simulink model "MagNoiseTest"  (R2022b)
settings: Solver=ode4  StartTime=0.0  StopTime=6000  FixedStep=dm.dt  RelTol=1e-3
InitFcn:
  | Tu = 210; %s
  | Wu   = 2*pi/Tu;
  | Zeta = 0.707;
  | SOFC = tf(Wu^2,[1 2*Zeta*Wu Wu^2]);
  | SOFD = c2d(SOFC, fsw.bdot_period);
undefined symbols (not defined in the file or in its folder): dm
libraries: aerolibtransform2 x1
settings Model: VariantFading=off  Creator=USER  LastModifiedBy=Jack-STK2

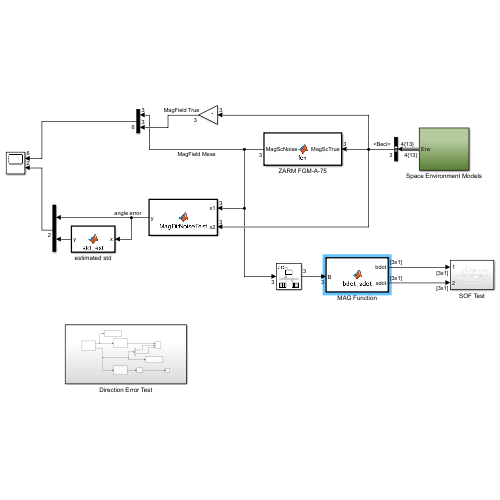
[thumbnail: Simulink's stored preview of the top-level diagram]
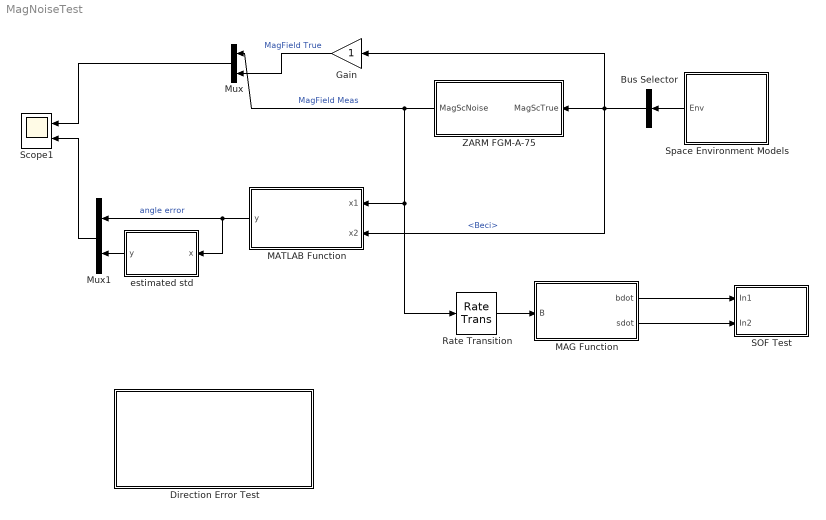
== system MagNoiseTest ==
  Bus Selector : BusSelector  OutputSignals=Beci
  Direction Error Test : Subsystem
  Gain : Gain
  MAG Function : MATLAB Function  TreatAsAtomicUnit=on
  MATLAB Function : MATLAB Function  TreatAsAtomicUnit=on
  Mux : Mux  Inputs=2
  Mux1 : Mux  Inputs=2
  Rate Transition : RateTransition  InitialCondition=zeros(3,1)  OutPortSampleTime=fsw.bdot_period
  SOF Test : Subsystem
  Scope1 : Scope  NumInputPorts=2
  Space Environment Models : Subsystem
  ZARM FGM-A-75 : MATLAB Function  TreatAsAtomicUnit=on
  estimated std : MATLAB Function  TreatAsAtomicUnit=on
  wires:
  Space Environment Models/1(Env) -> Bus Selector/1
  Bus Selector/1 -> ZARM FGM-A-75/1(MagScTrue), Gain/1, MATLAB Function/2(x2)  "<Beci>"
  ZARM FGM-A-75/1(MagScNoise) -> MATLAB Function/1(x1), Rate Transition/1, Mux/1  "MagField Meas"
  MATLAB Function/1(y) -> estimated std/1(x), Mux1/1  "angle error"
  Mux/1 -> Scope1/1
  Gain/1 -> Mux/2  "MagField True"
  estimated std/1(y) -> Mux1/2
  Mux1/1 -> Scope1/2
  Rate Transition/1 -> MAG Function/1(B)
  MAG Function/1(bdot) -> SOF Test/1(In1)
  MAG Function/2(sdot) -> SOF Test/2(In2)

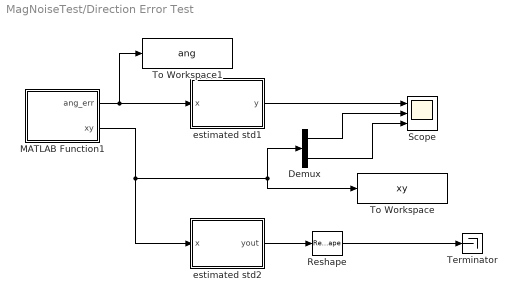
== system MagNoiseTest/Direction Error Test ==
  Demux : Demux  Outputs=2
  MATLAB Function1 : MATLAB Function  TreatAsAtomicUnit=on
  Reshape : Reshape
  Scope : Scope  NumInputPorts=3
  Terminator : Terminator
  To Workspace : ToWorkspace  VariableName=xy  SaveFormat=Timeseries  SampleTime=-1
      settings: Save2DSignal=2-D array (concatenate along first dimension)
  To Workspace1 : ToWorkspace  VariableName=ang  SaveFormat=Timeseries  SampleTime=-1
  estimated std1 : MATLAB Function  TreatAsAtomicUnit=on
  estimated std2 : MATLAB Function  TreatAsAtomicUnit=on
  wires:
  Demux/2 -> Scope/3
  MATLAB Function1/1(ang_err) -> To Workspace1/1, estimated std1/1(x)
  Demux/1 -> Scope/2
  estimated std2/1(yout) -> Reshape/1
  Reshape/1 -> Terminator/1
  MATLAB Function1/2(xy) -> Demux/1, To Workspace/1, estimated std2/1(x)
  estimated std1/1(y) -> Scope/1

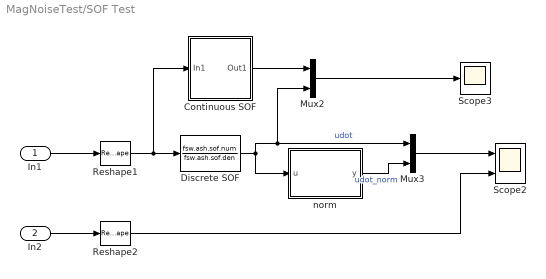
== system MagNoiseTest/SOF Test ==
  In1 : Inport
  In2 : Inport  Port=2
  Continuous SOF : Subsystem
  Discrete SOF : DiscreteTransferFcn  Numerator=fsw.ash.sof.num  Denominator=fsw.ash.sof.den
  Mux2 : Mux  Inputs=2
  Mux3 : Mux  Inputs=2
  Reshape1 : Reshape
  Reshape2 : Reshape
  Scope2 : Scope  NumInputPorts=2
  Scope3 : Scope
  norm : MATLAB Function  TreatAsAtomicUnit=on
  wires:
  Continuous SOF/1(Out1) -> Mux2/1
  Mux3/1 -> Scope2/1
  norm/1(y) -> Mux3/2  "udot_norm"
  Discrete SOF/1 -> norm/1(u), Mux2/2, Mux3/1  "udot"
  Mux2/1 -> Scope3/1
  Reshape1/1 -> Continuous SOF/1(In1), Discrete SOF/1
  Reshape2/1 -> Scope2/2
  In1/1 -> Reshape1/1
  In2/1 -> Reshape2/1

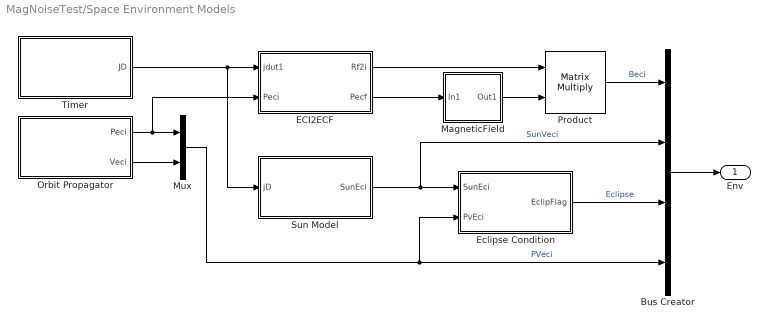
== system MagNoiseTest/Space Environment Models ==
  Bus Creator : BusCreator  Inputs=4
  ECI2ECF : MATLAB Function  TreatAsAtomicUnit=on
  Eclipse Condition : MATLAB Function  TreatAsAtomicUnit=on
  MagneticField : Subsystem
  Mux : Mux  Inputs=2
  "Orbit Propagator " : Subsystem
  Product : Product  Multiplication=Matrix(*)
  Sun Model : MATLAB Function  TreatAsAtomicUnit=on
  Timer : Subsystem
  Env : Outport  VectorParamsAs1DForOutWhenUnconnected=off
  wires:
  ECI2ECF/1(Rf2i) -> Product/1
  Product/1 -> Bus Creator/1  "Beci"
  "Orbit Propagator "/1(Peci) -> ECI2ECF/2(Peci), Mux/1
  "Orbit Propagator "/2(Veci) -> Mux/2
  Timer/1(JD) -> Sun Model/1(jD), ECI2ECF/1(jdut1)
  Mux/1 -> Eclipse Condition/2(PvEci), Bus Creator/4  "PVeci"
  Bus Creator/1 -> Env/1
  Sun Model/1(SunEci) -> Bus Creator/2, Eclipse Condition/1(SunEci)  "SunVeci"
  Eclipse Condition/1(EclipFlag) -> Bus Creator/3  "Eclipse"
  ECI2ECF/2(Pecf) -> MagneticField/1(In1)
  MagneticField/1(Out1) -> Product/2

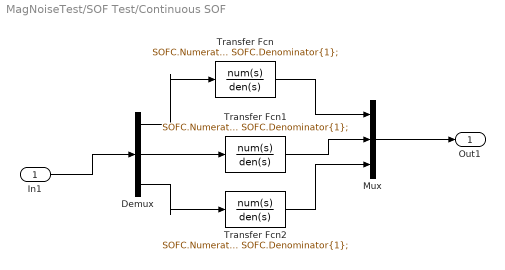
== system MagNoiseTest/SOF Test/Continuous SOF ==
  In1 : Inport
  Demux : Demux  Outputs=3
  Mux : Mux  Inputs=3
  Transfer Fcn : TransferFcn  Numerator=SOFC.Numerator{1}  Denominator=SOFC.Denominator{1};
  Transfer Fcn1 : TransferFcn  Numerator=SOFC.Numerator{1}  Denominator=SOFC.Denominator{1};
  Transfer Fcn2 : TransferFcn  Numerator=SOFC.Numerator{1}  Denominator=SOFC.Denominator{1};
  Out1 : Outport
  wires:
  In1/1 -> Demux/1
  Demux/1 -> Transfer Fcn/1
  Demux/2 -> Transfer Fcn1/1
  Demux/3 -> Transfer Fcn2/1
  Transfer Fcn/1 -> Mux/1
  Transfer Fcn1/1 -> Mux/2
  Transfer Fcn2/1 -> Mux/3
  Mux/1 -> Out1/1

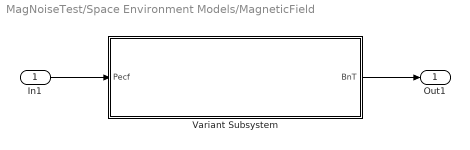
== system MagNoiseTest/Space Environment Models/MagneticField ==
  In1 : Inport
  Variant Subsystem : Subsystem  Variant=on
  Out1 : Outport
  wires:
  In1/1 -> Variant Subsystem/1(Pecf)
  Variant Subsystem/1(BnT) -> Out1/1

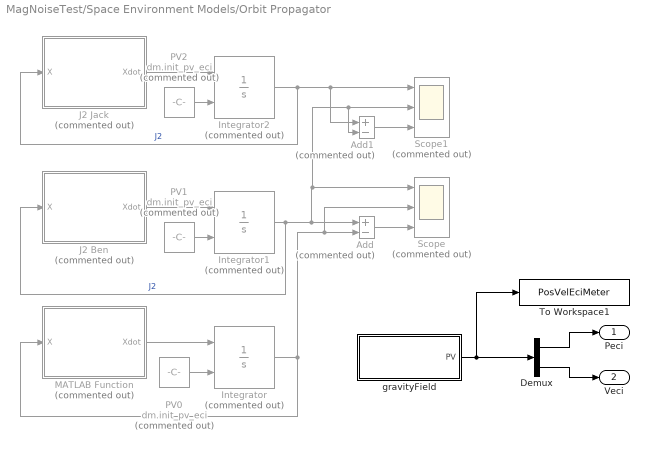
== system MagNoiseTest/Space Environment Models/Orbit Propagator  ==
  Add : Sum  Commented=on  Inputs=+-
  Add1 : Sum  Commented=on  Inputs=+-
  Demux : Demux  Outputs=2
  Integrator : Integrator  Commented=on  InitialConditionSource=external
  Integrator1 : Integrator  Commented=on  InitialConditionSource=external
  Integrator2 : Integrator  Commented=on  InitialConditionSource=external
  J2 Ben : MATLAB Function  Commented=on  TreatAsAtomicUnit=on
  J2 Jack : MATLAB Function  Commented=on  TreatAsAtomicUnit=on
  MATLAB Function : MATLAB Function  Commented=on  TreatAsAtomicUnit=on
  PV0 : Constant  Commented=on  Value=dm.init_pv_eci
  PV1 : Constant  Commented=on  Value=dm.init_pv_eci
  PV2 : Constant  Commented=on  Value=dm.init_pv_eci
  Scope : Scope  Commented=on  NumInputPorts=3
  Scope1 : Scope  Commented=on  NumInputPorts=3
  To Workspace1 : ToWorkspace  VariableName=PosVelEciMeter  SaveFormat=Timeseries  SampleTime=-1
  gravityField : Subsystem  Variant=on
  Peci : Outport  VectorParamsAs1DForOutWhenUnconnected=off
  Veci : Outport  Port=2  VectorParamsAs1DForOutWhenUnconnected=off
  wires:
  Demux/2 -> Veci/1
  MATLAB Function/1(Xdot) -> Integrator/1
  Integrator/1 -> Add/2, Scope/2, MATLAB Function/1(X)
  Demux/1 -> Peci/1
  PV0/1 -> Integrator/2
  PV1/1 -> Integrator1/2
  J2 Ben/1(Xdot) -> Integrator1/1
  Integrator1/1 -> J2 Ben/1(X), Add/1, Add1/2, Scope1/2, Scope/1  "J2"
  Add/1 -> Scope/3
  PV2/1 -> Integrator2/2
  J2 Jack/1(Xdot) -> Integrator2/1
  Integrator2/1 -> J2 Jack/1(X), Add1/1, Scope1/1  "J2"
  Add1/1 -> Scope1/3
  gravityField/1(PV) -> To Workspace1/1, Demux/1

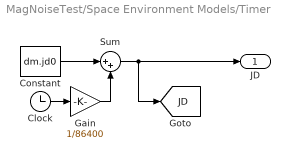
== system MagNoiseTest/Space Environment Models/Timer ==
  Clock : Clock
  Constant : Constant  Value=dm.jd0
  Gain : Gain  Gain=1/86400
  Sum : Sum  Inputs=|++
  JD : Outport  VectorParamsAs1DForOutWhenUnconnected=off
  tag scope: JD=global
  wires:
  Clock/1 -> Gain/1
  Gain/1 -> Sum/2
  Constant/1 -> Sum/1
  Sum/1 -> [JD], JD/1

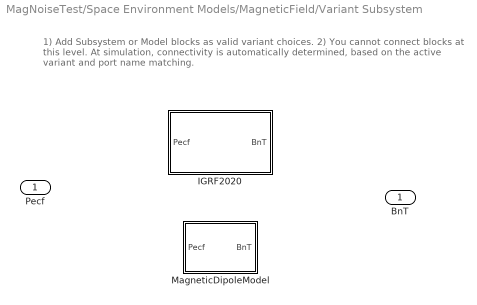
== system MagNoiseTest/Space Environment Models/MagneticField/Variant Subsystem ==
  note: 1) Add Subsystem or Model blocks as valid variant choices.
      | 2) You cannot connect blocks at this level. At simulation, connectivity is automatically
      | determined, based on the active variant and port name matching.
  Pecf : Inport
  IGRF2020 : Subsystem  VariantControl=M_IGRF
  MagneticDipoleModel : MATLAB Function  TreatAsAtomicUnit=on  VariantControl=M_DIPOLE
  BnT : Outport

== system MagNoiseTest/Space Environment Models/Orbit Propagator /gravityField ==
  note: 1) Add Subsystem or Model blocks as valid variant choices.
      | 2) You cannot connect blocks at this level. At simulation, connectivity is automatically
      | determined, based on the active variant and port name matching.
  J2 : Subsystem  VariantControl=G_J2
  TwoBodyRHS : Subsystem  VariantControl=G_TwoBody
  PV : Outport

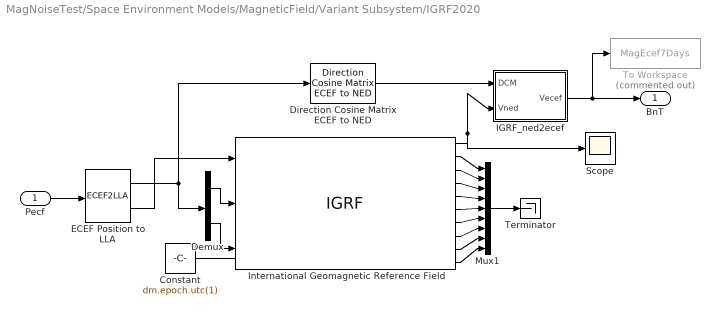
== system MagNoiseTest/Space Environment Models/MagneticField/Variant Subsystem/IGRF2020 ==
  Pecf : Inport
  Constant : Constant  Value=dm.epoch.utc(1)
  Demux : Demux  Outputs=2
  Direction Cosine Matrix ECEF to NED : aerolibtransform2/Direction Cosine Matrix ECEF to NED
  ECEF Position to LLA : ECEF2LLA  R=6378137
  IGRF_ned2ecef : MATLAB Function  TreatAsAtomicUnit=on
  International Geomagnetic Reference Field : IGRF  time_in=off  month=June  day=21  year=2023
      settings: AttributesFormatString=%<generation>
  Mux1 : Mux  Inputs=9
  Scope : Scope
  Terminator : Terminator
  To Workspace : ToWorkspace  Commented=on  VariableName=MagEcef7Days  SaveFormat=Timeseries  SampleTime=-1
  BnT : Outport  VectorParamsAs1DForOutWhenUnconnected=off
  wires:
  International Geomagnetic Reference Field/7 -> Mux1/6
  International Geomagnetic Reference Field/4 -> Mux1/3
  International Geomagnetic Reference Field/3 -> Mux1/2
  International Geomagnetic Reference Field/6 -> Mux1/5
  International Geomagnetic Reference Field/5 -> Mux1/4
  International Geomagnetic Reference Field/9 -> Mux1/8
  International Geomagnetic Reference Field/8 -> Mux1/7
  International Geomagnetic Reference Field/10 -> Mux1/9
  Pecf/1 -> ECEF Position to LLA/1
  Mux1/1 -> Terminator/1
  International Geomagnetic Reference Field/2 -> Mux1/1
  ECEF Position to LLA/1 -> Demux/1, Direction Cosine Matrix ECEF to NED/1
  ECEF Position to LLA/2 -> International Geomagnetic Reference Field/1
  Constant/1 -> ?
  Demux/1 -> International Geomagnetic Reference Field/2
  Demux/2 -> International Geomagnetic Reference Field/3
  Direction Cosine Matrix ECEF to NED/1 -> IGRF_ned2ecef/1(DCM)
  IGRF_ned2ecef/1(Vecef) -> To Workspace/1, BnT/1
  International Geomagnetic Reference Field/1 -> IGRF_ned2ecef/2(Vned), Scope/1

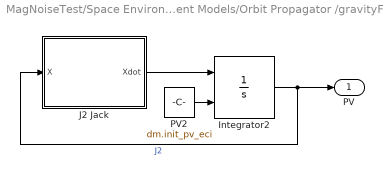
== system MagNoiseTest/Space Environment Models/Orbit Propagator /gravityField/J2 ==
  Integrator2 : Integrator  InitialConditionSource=external
  J2 Jack : MATLAB Function  TreatAsAtomicUnit=on
  PV2 : Constant  Value=dm.init_pv_eci
  PV : Outport
  wires:
  Integrator2/1 -> PV/1, J2 Jack/1(X)  "J2"
  J2 Jack/1(Xdot) -> Integrator2/1
  PV2/1 -> Integrator2/2

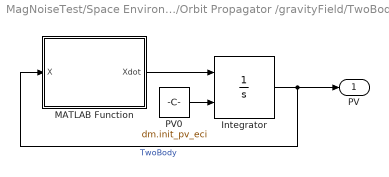
== system MagNoiseTest/Space Environment Models/Orbit Propagator /gravityField/TwoBodyRHS ==
  Integrator : Integrator  InitialConditionSource=external
  MATLAB Function : MATLAB Function  TreatAsAtomicUnit=on
  PV0 : Constant  Value=dm.init_pv_eci
  PV : Outport
  wires:
  Integrator/1 -> PV/1, MATLAB Function/1(X)  "TwoBody"
  MATLAB Function/1(Xdot) -> Integrator/1
  PV0/1 -> Integrator/2

== matlab function MagNoiseTest/Space Environment Models/Sun Model ==
  data: jD input; SunEci output
function SunEci = SunModel(jD)
T = JDCentury(jD);
lamda_mean     = rem(280.460+36000.771*T,360);
mean_anomaly   = rem(357.5291092+35999.05034*T,360);
lamda_ecliptic = lamda_mean+ 1.914666471*sind(mean_anomaly)...
                 + 0.019994643*sind(2*mean_anomaly);
% Obliquity of ecliptic
epsilon = 23.439291 -0.0130042*T;
SunEci  = [cosd(lamda_ecliptic);...
           cosd(epsilon)*sind(lamda_ecliptic);...
           sind(epsilon)*sind(lamda_ecliptic)];

== matlab function MagNoiseTest/Space Environment Models/MagneticField/Variant Subsystem/IGRF2020/IGRF_ned2ecef ==
  data: DCM input; Vecef output; Vned input
function Vecef = fcn(DCM,Vned)

Vecef = DCM'*Vned;

== matlab function MagNoiseTest/Space Environment Models/ECI2ECF ==
  data: Rf2i output; jdut1 input; Pecf output; Peci input
%% ECI to ECEF Transformation
function [Rf2i, Pecf]  = ECI2ECF(jdut1, Peci)
Ri2f  = R3(JD2GMST(jdut1));
Pecf  = Ri2f*Peci; %in m
Rf2i  = Ri2f';

== matlab function MagNoiseTest/Space Environment Models/Orbit Propagator /J2 Ben ==
  data: X input; Xdot output; dm parameter
function Xdot = J2(X, dm)

r = X(1:3);
v = X(4:6);
J2 = 0.484165143790815D-03*(5)^0.5;
GMe = 3.986004418e14;                % m^3*s^-2
Re = 6378137;                        % earth radius, m
k_1_2 = -GMe/norm(r)^3 * (1+ 1.5 *J2* (Re/norm(r))^2 * (1 - 5* (r(3)/norm(r))^2) );
k_3 = -GMe/norm(r)^3 * (1+ 1.5 *J2* (Re/norm(r))^2 * (3 - 5* (r(3)/norm(r))^2) );
a = [k_1_2*r(1); k_1_2*r(2); k_3*r(3)];
Xdot=[v; a];

% Re   = 6378137.00;%m
% mu_e = 3.986004418e14;%3.986004418e14;
% 
% p = X(1:3);
% v = X(4:6);
% R = norm(p);
% 
% 
% J2 = 0.001082626173852;%0.001082626173852;% C20_bar = -0.484165143790815D-03 from EGM2008
% %0.001082626683553151; STK
%      
% ReOverR_2 = (Re/R)^2;
% sinphi_2   = (p(3)/R)^2;
% muOverR_3 = mu_e/R^3;
% vdot=[-muOverR_3*(1+1.5*J2*ReOverR_2*(1-5*sinphi_2));...
%       -muOverR_3*(1+1.5*J2*ReOverR_2*(1-5*sinphi_2));...
%       -muOverR_3*(1+1.5*J2*ReOverR_2*(3-5*sinphi_2))].*p;
%      
% Xdot=[v; vdot];

== matlab function MagNoiseTest/Space Environment Models/Orbit Propagator /J2 Jack ==
  data: X input; Xdot output; dm parameter
function Xdot = J2(X, dm)

Re   = 6378137.00;%m
mu_e = 3.986004418e14;%3.986004418e14;

p = X(1:3);
v = X(4:6);
R = norm(p);


J2 = 0.001082626173852;%0.001082626173852;% C20_bar = -0.484165143790815D-03 from EGM2008
%0.001082626683553151; STK
     
ReOverR_2 = (Re/R)^2;
sinphi_2   = (p(3)/R)^2;
muOverR_3 = mu_e/R^3;
vdot=[-muOverR_3*(1+1.5*J2*ReOverR_2*(1-5*sinphi_2));...
      -muOverR_3*(1+1.5*J2*ReOverR_2*(1-5*sinphi_2));...
      -muOverR_3*(1+1.5*J2*ReOverR_2*(3-5*sinphi_2))].*p;
     
Xdot=[v; vdot];

== matlab function MagNoiseTest/Space Environment Models/Orbit Propagator /gravityField/TwoBodyRHS/MATLAB Function ==
  data: X input; Xdot output; dm parameter
function Xdot = TwoBodyRHS(X, dm)

r = X(1:3);
v = X(4:6);
Xdot=[v; -(dm.mu_e*r/norm(r)^3)];

== matlab function MagNoiseTest/Space Environment Models/Orbit Propagator /gravityField/J2/J2 Jack ==
  data: X input; Xdot output; dm parameter
function Xdot = J2(X, dm)

Re   = 6378137.00;%m
mu_e = 3.986004418e14;%3.986004418e14;

p = X(1:3);
v = X(4:6);
R = norm(p);


J2 = 0.001082626173852;%0.001082626173852;% C20_bar = -0.484165143790815D-03 from EGM2008
%0.001082626683553151; STK
     
ReOverR_2 = (Re/R)^2;
sinphi_2   = (p(3)/R)^2;
muOverR_3 = mu_e/R^3;
vdot=[-muOverR_3*(1+1.5*J2*ReOverR_2*(1-5*sinphi_2));...
      -muOverR_3*(1+1.5*J2*ReOverR_2*(1-5*sinphi_2));...
      -muOverR_3*(1+1.5*J2*ReOverR_2*(3-5*sinphi_2))].*p;
     
Xdot=[v; vdot];

== matlab function MagNoiseTest/Space Environment Models/Orbit Propagator /MATLAB Function ==
  data: X input; Xdot output; dm parameter
function Xdot = TwoBodyRHS(X, dm)

r = X(1:3);
v = X(4:6);
Xdot=[v; -(dm.mu_e*r/norm(r)^3)];

== matlab function MagNoiseTest/Space Environment Models/MagneticField/Variant Subsystem/MagneticDipoleModel ==
  data: Pecf input; BnT output; dm parameter
function BnT = MagDipole(Pecf, dm)

BnT = MagneticDipole(Pecf, dm.mpm);

== matlab function MagNoiseTest/MATLAB Function ==
  data: x1 input; y output; x2 input
function y = MagDirNoiseTest(x1, x2)


x1_dir = x1/norm(x1);
x2_dir = x2/norm(x2);
y = acosd(dot(x1_dir,x2_dir));

== matlab function MagNoiseTest/ZARM FGM-A-75 ==
  settings: updateMethod=DISCRETE
  data: MagScTrue input; MagScNoise output size=3; dm parameter
function MagScNoise = fcn(MagScTrue, dm)

mag_norm_ture = norm(MagScTrue);
if abs(mag_norm_ture-eps) < 10*eps
    MagScNoise = MagScTrue;
    return;
end
mag_dir_true  = MagScTrue/mag_norm_ture;

%% add direction noise
xy            = dm.mag_mdl.ang_err*randn(2,1)/2;
q_dist        = [sqrt(1-xy'*xy); xy; 0];
mag_dir_dist  = QMul(QInv(q_dist),QMul([0;mag_dir_true],q_dist));

%% add magnitude noise
mag_norm_dist = mag_norm_ture*(1 + dm.mag_mdl.norm_err*randn(1,1));
mag_dist      = mag_dir_dist(2:4)*mag_norm_dist;

%% add linear, offset, noise
MagScNoise    = mag_dist + dm.mag_mdl.noise * randn(3,1)...
                         + dm.mag_mdl.linerity_err * randn(3,1)...
                         + dm.mag_mdl.offset_err * randn(3,1);
end

== matlab function MagNoiseTest/estimated std ==
  settings: updateMethod=DISCRETE
  data: x input; y output
function y = std_est(x)

persistent mk_1 sk_1 n
if isempty(mk_1)
    mk_1 =x(1);
    sk_1 = 0;
    n = 2;
end

mk    = (n-1)/n*mk_1+x/n;
sk    = sk_1+(n-1)/n*(x-mk_1)^2;
vark  = sk/(n);
y     = sqrt(vark);
sk_1  = sk;
mk_1  = mk;
n = n+1;

== matlab function MagNoiseTest/Direction Error Test/MATLAB Function1 ==
  data: ang_err output; dm parameter; xy output size=2
function [ang_err,xy] = fcn(dm)


% rdn_dir = [randn(2,1);0];        % only for x and y axis
% rdn_dir = rdn_dir/norm(rdn_dir);
% thet_dist = dm.mag_mdl.ang_err*randn(1,1)/2*1.549; %half noise
% fct = 1.549;
xy=dm.mag_mdl.ang_err*randn(2,1)/2;
q_dist = [sqrt(1-xy'*xy); xy; 0];
% q_dist = [cos(thet_dist); rdn_dir*sin(thet_dist)];

% mag_dir_dist = QMul([1;0;0;0],q_dist);
mag_dir_dist = QMul(QInv(q_dist),QMul([0;0;0;1],q_dist));
ang_err = acosd(mag_dir_dist(4));
xy = [mag_dir_dist(2); mag_dir_dist(3)];

== matlab function MagNoiseTest/Direction Error Test/estimated std1 ==
  settings: updateMethod=DISCRETE
  data: x input; y output
function y = std_est(x)

persistent mk_1 sk_1 n
if isempty(mk_1)
    mk_1 = x;
    sk_1 = 0;
    n = 2;
end

mk    = mk_1*((n-1)/n) + x/n;
sk    = sk_1+(x-mk_1).^2*((n-1)/n);
vark  = sk/(n);
y     = sqrt(vark);
sk_1  = sk;
mk_1  = mk;
n = n+1;

== matlab function MagNoiseTest/Direction Error Test/estimated std2 ==
  settings: updateMethod=DISCRETE
  data: x input; yout output
function yout = std_est(x)

persistent mk_1 sk_1 n

if isempty(mk_1)
     mk_1 = x;
     sk_1 = zeros(length(x),1);
     n = 2;
end

mk    = mk_1*((n-1)/n) + x/n;
sk    = sk_1+(x-mk_1).^2*((n-1)/n);
vark  = sk/(n);
yout     = sqrt(vark);

sk_1  = sk;
mk_1  = mk;
n = n+1;

== matlab function MagNoiseTest/MAG Function ==
  data: B input; fsw parameter; bdot output; sdot output
function [bdot, sdot] =  bdot_sdot(B, fsw)

persistent b_1
B_NORM = norm(B);
b      = B/B_NORM;
if isempty(b_1)
    b_1 = b;
end

bdot = (b-b_1)/fsw.bdot_period;
sdot = (bdot-b*(b'*bdot))/B_NORM;

b_1 = b;

== matlab function MagNoiseTest/SOF Test/norm ==
  data: u input; y output
function y = fcn(u)

y = norm(u);

== matlab function MagNoiseTest/Space Environment Models/Eclipse Condition ==
  data: SunEci input; EclipFlag output; PvEci input
function EclipFlag  = Eclipse(SunEci, PvEci)
Dp = -PvEci(1:3)*1e-3;  % earth vector in Km
Rp = 6378.137;          % earth radius in km
Rs = 6.9599e5;          % solar photosphere radius in km
S  = 1.49597870e8;      % astronomical unit in km
C  = 1.385e6;           % size of earth shadow cone
Ds = (S.*SunEci + Dp);  % vector from S/C to the Sun

DsNorm = norm(Ds);
DpNorm = norm(Dp);
rho_s  = asind(Rs/DsNorm);
rho_p  = asind(Rp/DpNorm);
theta  = acosd(dot(Ds, Dp) / (DsNorm * DpNorm));
if ( theta < (rho_p - rho_s) && DsNorm > S && (S + C) > DsNorm)
    EclipFlag = 1;
else
	EclipFlag = 0;
end
